simulink model "pf_sim"  (R2018b)
settings: Solver=FixedStepAuto  StartTime=0.0  StopTime=400  FixedStep=0.0001  RelTol=1e-5  EnableMultiTasking=on
StopFcn:
  | %e_unicycle_3d_trefoil_plot
libraries: simulink x4
settings Model: Creator=winston  LastModifiedBy=winston
settings SolverCC: AutoInsertRateTranBlk=on
settings DataIOCC: SaveOutput=off  SignalLogging=off  DSMLogging=off  SaveTime=off
settings OptimizationCC: LifeSpan=inf
settings DebuggingCC: AllowSymbolicDim=off  SFUnexpectedBacktrackingDiag=warning  SFNoUnconditionalDefaultTransitionDiag=warning  SFExecutionAtInitializationDiag=none  UnderSpecifiedDimensionMsg=warning
settings ModelReferenceCC: PropagateSignalLabelsOutOfModel=off
settings SFSimCC: SimUseLocalCustomCode=off
settings RTWCC: RTWUseLocalCustomCode=off
settings CodeAppCC: StateflowObjectComments=on
settings GRTTargetCC: TargetLangStandard=C89/C90 (ANSI)
settings ConfigComp: CovMetricSettings=dw  CovHtmlReporting=on  CovSaveCumulativeToWorkspaceVar=on  CovSaveSingleToWorkspaceVar=on  CovExternalEMLEnable=off

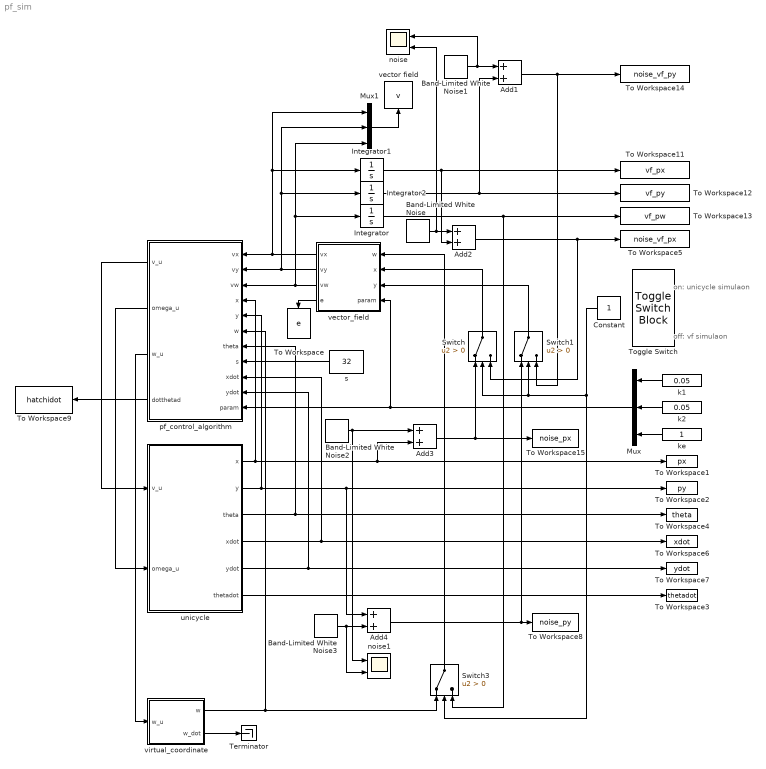
== system pf_sim ==
  note: off: vf simulaon
  note: on: unicycle simulaon
  Add{1..4} (4 alike) : Sum
  Band-Limited White Noise : simulink/Sources/Band-Limited White Noise  Cov=10  Ts=0.1  seed=[23341]
  Band-Limited White Noise1 : simulink/Sources/Band-Limited White Noise  Cov=10  Ts=0.1  seed=[241]
  Band-Limited White Noise2 : simulink/Sources/Band-Limited White Noise  Cov=10  Ts=0.1  seed=[23341]
  Band-Limited White Noise3 : simulink/Sources/Band-Limited White Noise  Cov=10  Ts=0.1  seed=[241]
  Constant : Constant
  Integrator : Integrator  InitialCondition=47
  Integrator1 : Integrator  InitialCondition=300
  Integrator2 : Integrator  InitialCondition=300
  Mux : Mux  Inputs=3
  Mux1 : Mux  Inputs=3
  Switch : Switch  Criteria=u2 > Threshold
  Switch1 : Switch  Criteria=u2 > Threshold
  Switch3 : Switch  Criteria=u2 > Threshold
  Terminator : Terminator
  To Workspace : ToWorkspace  VariableName=e  SaveFormat=Timeseries  SampleTime=-1
  To Workspace1 : ToWorkspace  VariableName=px  SampleTime=-1
  To Workspace11 : ToWorkspace  VariableName=vf_px  SampleTime=-1
  To Workspace12 : ToWorkspace  VariableName=vf_py  SampleTime=-1
  To Workspace13 : ToWorkspace  VariableName=vf_pw  SampleTime=-1
  To Workspace14 : ToWorkspace  VariableName=noise_vf_py  SampleTime=-1
  To Workspace15 : ToWorkspace  VariableName=noise_px  SampleTime=-1
  To Workspace2 : ToWorkspace  VariableName=py  SampleTime=-1
  To Workspace3 : ToWorkspace  VariableName=thetadot  SampleTime=-1
  To Workspace4 : ToWorkspace  VariableName=theta  SampleTime=-1
  To Workspace5 : ToWorkspace  VariableName=noise_vf_px  SampleTime=-1
  To Workspace6 : ToWorkspace  VariableName=xdot  SampleTime=-1
  To Workspace7 : ToWorkspace  VariableName=ydot  SampleTime=-1
  To Workspace8 : ToWorkspace  VariableName=noise_py  SampleTime=-1
  To Workspace9 : ToWorkspace  VariableName=hatchidot  SampleTime=-1
  Toggle Switch : ToggleSwitchBlock  WebBlockId=86
      settings: Values={{'Off', 'On'}, [-1 1]}
  k1 : Constant  Value=0.05
  k2 : Constant  Value=0.05
  ke : Constant
  noise : Scope  NumInputPorts=2
  noise1 : Scope  NumInputPorts=2
  pf_control_algorithm : MATLAB Function  TreatAsAtomicUnit=on
  s : Constant  Value=32
  unicycle : Subsystem  mask{x0=300, y0=300, theta0=0}
      mask prompts: x0 "x(0)"; y0 "y(0)"; theta0 "theta(0)"
  vector field : ToWorkspace  VariableName=v  SaveFormat=Timeseries  SampleTime=-1
  vector_field : Subsystem
  virtual_coordinate : Subsystem  mask{w0=0}
      mask prompts: w0 "w(0)"
  wires:
  unicycle/1(x) -> pf_control_algorithm/4(x), Add3/2, To Workspace1/1
  unicycle/2(y) -> pf_control_algorithm/5(y), To Workspace2/1, Add4/1
  unicycle/3(theta) -> pf_control_algorithm/7(theta), To Workspace4/1
  unicycle/4(xdot) -> pf_control_algorithm/9(xdot), To Workspace6/1
  unicycle/5(ydot) -> pf_control_algorithm/10(ydot), To Workspace7/1
  Integrator/1 -> Switch3/3, To Workspace13/1
  Mux/1 -> pf_control_algorithm/11(param), vector_field/4(param)
  pf_control_algorithm/1(v_u) -> unicycle/1(v_u)
  pf_control_algorithm/2(omega_u) -> unicycle/2(omega_u)
  Integrator1/1 -> To Workspace11/1, Add2/2
  k1/1 -> Mux/1
  k2/1 -> Mux/2
  ke/1 -> Mux/3
  Mux1/1 -> vector field/1
  Constant/1 -> Switch/2, Switch1/2, Switch3/2
  vector_field/1(vx) -> pf_control_algorithm/1(vx), Integrator1/1, Mux1/1
  vector_field/3(vw) -> pf_control_algorithm/3(vw), Mux1/3, Integrator/1
  vector_field/2(vy) -> pf_control_algorithm/2(vy), Integrator2/1, Mux1/2
  Switch/1 -> vector_field/2(x)
  Switch1/1 -> vector_field/3(y)
  vector_field/4(e) -> To Workspace/1
  pf_control_algorithm/3(w_u) -> virtual_coordinate/1(w_u)
  virtual_coordinate/1(w) -> pf_control_algorithm/6(w), Switch3/1
  Switch3/1 -> vector_field/1(w)
  s/1 -> pf_control_algorithm/8(s)
  unicycle/6(thetadot) -> To Workspace3/1
  pf_control_algorithm/4(dotthetad) -> To Workspace9/1
  Add1/1 -> To Workspace14/1, Switch1/3
  Band-Limited White Noise1/1 -> noise/1, Add1/1
  Integrator2/1 -> To Workspace12/1, Add1/2
  Band-Limited White Noise/1 -> noise/2, Add2/1
  Add2/1 -> Switch/3, To Workspace5/1
  Band-Limited White Noise2/1 -> Add3/1, noise1/1
  Add3/1 -> Switch/1, To Workspace15/1
  Band-Limited White Noise3/1 -> noise1/2, Add4/2
  Add4/1 -> Switch1/1, To Workspace8/1
  virtual_coordinate/2(w_dot) -> Terminator/1

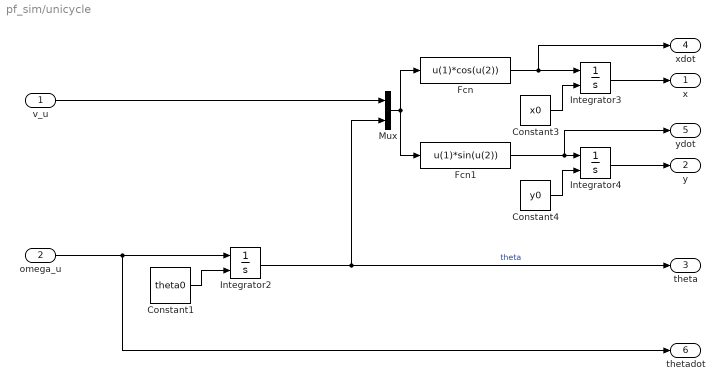
== system pf_sim/unicycle ==
  v_u : Inport
  omega_u : Inport  Port=2
  Constant1 : Constant  Value=theta0
  Constant3 : Constant  Value=x0
  Constant4 : Constant  Value=y0
  Fcn : Fcn  Expr=u(1)*cos(u(2))
  Fcn1 : Fcn  Expr=u(1)*sin(u(2))
  Integrator2 : Integrator  InitialConditionSource=external
  Integrator3 : Integrator  InitialConditionSource=external
  Integrator4 : Integrator  InitialConditionSource=external
  Mux : Mux  Inputs=2
  x : Outport
  y : Outport  Port=2
  theta : Outport  Port=3
  xdot : Outport  Port=4
  ydot : Outport  Port=5
  thetadot : Outport  Port=6
  wires:
  v_u/1 -> Mux/1
  Integrator2/1 -> theta/1, Mux/2  "theta"
  Mux/1 -> Fcn/1, Fcn1/1
  Fcn/1 -> xdot/1, Integrator3/1
  Fcn1/1 -> ydot/1, Integrator4/1
  Integrator3/1 -> x/1
  Integrator4/1 -> y/1
  Constant1/1 -> Integrator2/2
  Constant3/1 -> Integrator3/2
  Constant4/1 -> Integrator4/2
  omega_u/1 -> thetadot/1, Integrator2/1

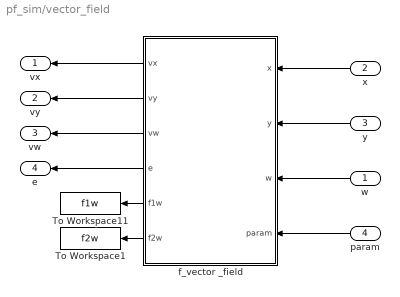
== system pf_sim/vector_field ==
  w : Inport
  x : Inport  Port=2
  y : Inport  Port=3
  param : Inport  Port=4
  To Workspace1 : ToWorkspace  VariableName=f2w  SampleTime=-1
  To Workspace11 : ToWorkspace  VariableName=f1w  SampleTime=-1
  f_vector _field : MATLAB Function  TreatAsAtomicUnit=on
  vx : Outport
  vy : Outport  Port=2
  vw : Outport  Port=3
  e : Outport  Port=4
  wires:
  y/1 -> f_vector _field/2(y)
  f_vector _field/1(vx) -> vx/1
  w/1 -> f_vector _field/3(w)
  f_vector _field/4(e) -> e/1
  f_vector _field/2(vy) -> vy/1
  x/1 -> f_vector _field/1(x)
  param/1 -> f_vector _field/4(param)
  f_vector _field/6(f2w) -> To Workspace1/1
  f_vector _field/5(f1w) -> To Workspace11/1
  f_vector _field/3(vw) -> vw/1

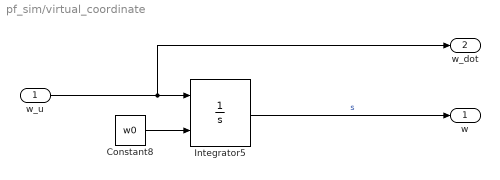
== system pf_sim/virtual_coordinate ==
  w_u : Inport
  Constant8 : Constant  Value=w0
  Integrator5 : Integrator  InitialConditionSource=external
  w : Outport
  w_dot : Outport  Port=2
  wires:
  Constant8/1 -> Integrator5/2
  w_u/1 -> w_dot/1, Integrator5/1
  Integrator5/1 -> w/1  "s"

== matlab function pf_sim/pf_control_algorithm ==
  data: vx input; vy input; vw input; v_u output; omega_u output; w_u output; x input; y input; w input; theta input; s input; xdot input; ydot input; param input; dotthetad output
function [v_u, omega_u, w_u, dotthetad] = fcn(vx, vy, vw, x, y, w, theta, s, xdot, ydot, param)
k1 = param(1); k2 = param(2); ke = param(3);

E = [0, -1; 1, 0];
chi = [vx; vy; vw];
hatchi = chi/norm(chi);
hatchip = hatchi(1:2);
h = [cos(theta); sin(theta)];
g = s * hatchip;
hatg = g / norm(g);
wdot = s*hatchi(3);            % speed in the virtual coordinate w

xidot=[xdot; ydot; wdot];   % note that here we should put the virtual speed 
                            % wdot rather than the acutal zdot!!!
                            
Jg = [ (s*(15*sin((3*w)/50 + 1/10) - k1*(250*cos((3*w)/50 + 1/10) - x + 600))*(2*k1*(15*sin((3*w)/50 + 1/10) - k1*(250*cos((3*w)/50 + 1/10) - x + 600)) - 30*k1*sin((3*w)/50 + 1/10)*(15*k1*sin((3*w)/50 + 1/10)*(250*cos((3*w)/50 + 1/10) - x + 600) + 20*k2*sin((2*w)/25 + 7/10)*(250*cos((2*w)/25 + 7/10) - y + 350) + 1)))/(2*((15*k1*sin((3*w)/50 + 1/10)*(250*cos((3*w)/50 + 1/10) - x + 600) + 20*k2*sin((2*w)/25 + 7/10)*(250*cos((2*w)/25 + 7/10) - y + 350) + 1)^2 + (15*sin((3*w)/50 + 1/10) - k1*(250*cos((3*w)/50 + 1/10) - x + 600))^2 + (20*sin((2*w)/25 + 7/10) - k2*(250*cos((2*w)/25 + 7/10) - y + 350))^2)^(3/2)) - (k1*s)/((15*k1*sin((3*w)/50 + 1/10)*(250*cos((3*w)/50 + 1/10) - x + 600) + 20*k2*sin((2*w)/25 + 7/10)*(250*cos((2*w)/25 + 7/10) - y + 350) + 1)^2 + (15*sin((3*w)/50 + 1/10) - k1*(250*cos((3*w)/50 + 1/10) - x + 600))^2 + (20*sin((2*w)/25 + 7/10) - k2*(250*cos((2*w)/25 + 7/10) - y + 350))^2)^(1/2),                                                                                                                                                                                                                                                                                                            (s*(15*sin((3*w)/50 + 1/10) - k1*(250*cos((3*w)/50 + 1/10) - x + 600))*(2*k2*(20*sin((2*w)/25 + 7/10) - k2*(250*cos((2*w)/25 + 7/10) - y + 350)) - 40*k2*sin((2*w)/25 + 7/10)*(15*k1*sin((3*w)/50 + 1/10)*(250*cos((3*w)/50 + 1/10) - x + 600) + 20*k2*sin((2*w)/25 + 7/10)*(250*cos((2*w)/25 + 7/10) - y + 350) + 1)))/(2*((15*k1*sin((3*w)/50 + 1/10)*(250*cos((3*w)/50 + 1/10) - x + 600) + 20*k2*sin((2*w)/25 + 7/10)*(250*cos((2*w)/25 + 7/10) - y + 350) + 1)^2 + (15*sin((3*w)/50 + 1/10) - k1*(250*cos((3*w)/50 + 1/10) - x + 600))^2 + (20*sin((2*w)/25 + 7/10) - k2*(250*cos((2*w)/25 + 7/10) - y + 350))^2)^(3/2)), (s*(15*sin((3*w)/50 + 1/10) - k1*(250*cos((3*w)/50 + 1/10) - x + 600))*(2*(15*sin((3*w)/50 + 1/10) - k1*(250*cos((3*w)/50 + 1/10) - x + 600))*((9*cos((3*w)/50 + 1/10))/10 + 15*k1*sin((3*w)/50 + 1/10)) - 2*(15*k1*sin((3*w)/50 + 1/10)*(250*cos((3*w)/50 + 1/10) - x + 600) + 20*k2*sin((2*w)/25 + 7/10)*(250*cos((2*w)/25 + 7/10) - y + 350) + 1)*(400*k2*sin((2*w)/25 + 7/10)^2 + 225*k1*sin((3*w)/50 + 1/10)^2 - (9*k1*cos((3*w)/50 + 1/10)*(250*cos((3*w)/50 + 1/10) - x + 600))/10 - (8*k2*cos((2*w)/25 + 7/10)*(250*cos((2*w)/25 + 7/10) - y + 350))/5) + 2*(20*sin((2*w)/25 + 7/10) - k2*(250*cos((2*w)/25 + 7/10) - y + 350))*((8*cos((2*w)/25 + 7/10))/5 + 20*k2*sin((2*w)/25 + 7/10))))/(2*((15*k1*sin((3*w)/50 + 1/10)*(250*cos((3*w)/50 + 1/10) - x + 600) + 20*k2*sin((2*w)/25 + 7/10)*(250*cos((2*w)/25 + 7/10) - y + 350) + 1)^2 + (15*sin((3*w)/50 + 1/10) - k1*(250*cos((3*w)/50 + 1/10) - x + 600))^2 + (20*sin((2*w)/25 + 7/10) - k2*(250*cos((2*w)/25 + 7/10) - y + 350))^2)^(3/2)) - (s*((9*cos((3*w)/50 + 1/10))/10 + 15*k1*sin((3*w)/50 + 1/10)))/((15*k1*sin((3*w)/50 + 1/10)*(250*cos((3*w)/50 + 1/10) - x + 600) + 20*k2*sin((2*w)/25 + 7/10)*(250*cos((2*w)/25 + 7/10) - y + 350) + 1)^2 + (15*sin((3*w)/50 + 1/10) - k1*(250*cos((3*w)/50 + 1/10) - x + 600))^2 + (20*sin((2*w)/25 + 7/10) - k2*(250*cos((2*w)/25 + 7/10) - y + 350))^2)^(1/2);
                                                                                                                                                                                                                                                                                                            (s*(20*sin((2*w)/25 + 7/10) - k2*(250*cos((2*w)/25 + 7/10) - y + 350))*(2*k1*(15*sin((3*w)/50 + 1/10) - k1*(250*cos((3*w)/50 + 1/10) - x + 600)) - 30*k1*sin((3*w)/50 + 1/10)*(15*k1*sin((3*w)/50 + 1/10)*(250*cos((3*w)/50 + 1/10) - x + 600) + 20*k2*sin((2*w)/25 + 7/10)*(250*cos((2*w)/25 + 7/10) - y + 350) + 1)))/(2*((15*k1*sin((3*w)/50 + 1/10)*(250*cos((3*w)/50 + 1/10) - x + 600) + 20*k2*sin((2*w)/25 + 7/10)*(250*cos((2*w)/25 + 7/10) - y + 350) + 1)^2 + (15*sin((3*w)/50 + 1/10) - k1*(250*cos((3*w)/50 + 1/10) - x + 600))^2 + (20*sin((2*w)/25 + 7/10) - k2*(250*cos((2*w)/25 + 7/10) - y + 350))^2)^(3/2)), (s*(20*sin((2*w)/25 + 7/10) - k2*(250*cos((2*w)/25 + 7/10) - y + 350))*(2*k2*(20*sin((2*w)/25 + 7/10) - k2*(250*cos((2*w)/25 + 7/10) - y + 350)) - 40*k2*sin((2*w)/25 + 7/10)*(15*k1*sin((3*w)/50 + 1/10)*(250*cos((3*w)/50 + 1/10) - x + 600) + 20*k2*sin((2*w)/25 + 7/10)*(250*cos((2*w)/25 + 7/10) - y + 350) + 1)))/(2*((15*k1*sin((3*w)/50 + 1/10)*(250*cos((3*w)/50 + 1/10) - x + 600) + 20*k2*sin((2*w)/25 + 7/10)*(250*cos((2*w)/25 + 7/10) - y + 350) + 1)^2 + (15*sin((3*w)/50 + 1/10) - k1*(250*cos((3*w)/50 + 1/10) - x + 600))^2 + (20*sin((2*w)/25 + 7/10) - k2*(250*cos((2*w)/25 + 7/10) - y + 350))^2)^(3/2)) - (k2*s)/((15*k1*sin((3*w)/50 + 1/10)*(250*cos((3*w)/50 + 1/10) - x + 600) + 20*k2*sin((2*w)/25 + 7/10)*(250*cos((2*w)/25 + 7/10) - y + 350) + 1)^2 + (15*sin((3*w)/50 + 1/10) - k1*(250*cos((3*w)/50 + 1/10) - x + 600))^2 + (20*sin((2*w)/25 + 7/10) - k2*(250*cos((2*w)/25 + 7/10) - y + 350))^2)^(1/2),  (s*(20*sin((2*w)/25 + 7/10) - k2*(250*cos((2*w)/25 + 7/10) - y + 350))*(2*(15*sin((3*w)/50 + 1/10) - k1*(250*cos((3*w)/50 + 1/10) - x + 600))*((9*cos((3*w)/50 + 1/10))/10 + 15*k1*sin((3*w)/50 + 1/10)) - 2*(15*k1*sin((3*w)/50 + 1/10)*(250*cos((3*w)/50 + 1/10) - x + 600) + 20*k2*sin((2*w)/25 + 7/10)*(250*cos((2*w)/25 + 7/10) - y + 350) + 1)*(400*k2*sin((2*w)/25 + 7/10)^2 + 225*k1*sin((3*w)/50 + 1/10)^2 - (9*k1*cos((3*w)/50 + 1/10)*(250*cos((3*w)/50 + 1/10) - x + 600))/10 - (8*k2*cos((2*w)/25 + 7/10)*(250*cos((2*w)/25 + 7/10) - y + 350))/5) + 2*(20*sin((2*w)/25 + 7/10) - k2*(250*cos((2*w)/25 + 7/10) - y + 350))*((8*cos((2*w)/25 + 7/10))/5 + 20*k2*sin((2*w)/25 + 7/10))))/(2*((15*k1*sin((3*w)/50 + 1/10)*(250*cos((3*w)/50 + 1/10) - x + 600) + 20*k2*sin((2*w)/25 + 7/10)*(250*cos((2*w)/25 + 7/10) - y + 350) + 1)^2 + (15*sin((3*w)/50 + 1/10) - k1*(250*cos((3*w)/50 + 1/10) - x + 600))^2 + (20*sin((2*w)/25 + 7/10) - k2*(250*cos((2*w)/25 + 7/10) - y + 350))^2)^(3/2)) - (s*((8*cos((2*w)/25 + 7/10))/5 + 20*k2*sin((2*w)/25 + 7/10)))/((15*k1*sin((3*w)/50 + 1/10)*(250*cos((3*w)/50 + 1/10) - x + 600) + 20*k2*sin((2*w)/25 + 7/10)*(250*cos((2*w)/25 + 7/10) - y + 350) + 1)^2 + (15*sin((3*w)/50 + 1/10) - k1*(250*cos((3*w)/50 + 1/10) - x + 600))^2 + (20*sin((2*w)/25 + 7/10) - k2*(250*cos((2*w)/25 + 7/10) - y + 350))^2)^(1/2)];
dotthetad = -1/norm(g)*transpose(hatg)*E*Jg*xidot;           
omega_u = dotthetad - ke*transpose(h)*E*hatg;      

w_u = wdot;
v_u = s*norm(hatchip);

== matlab function pf_sim/vector_field/f_vector _field ==
  data: vx output; vy output; vw output; e output; x input; y input; w input; param input; f1w output; f2w output
function [vx, vy, vw, e, f1w, f2w] = fcn(x, y, w, param)

k1 = param(1); k2 = param(2); 
e1 = x - 250*cos((3*w)/50 + 1/10) - 600;
e2 = y - 250*cos((2*w)/25 + 7/10) - 350;
f1w = x - e1;
f2w = y - e2;

n1 = [        1;
              0;
   15*sin((3*w)/50 + 1/10)];
n2 = [        0;
              1;
 20*sin((2*w)/25 + 7/10)];

nke = k1*e1*n1+k2*e2*n2;

v = cross(n1,n2) - nke;     % vector field

vx = v(1);
vy = v(2);
vw = v(3);
e = [e1; e2];
